simulink model "Vehicle_Model_Controller_Mar18"  (R2020b)
settings: Solver=VariableStepAuto  StartTime=0.0  StopTime=20  FixedStep=0.015  MaxStep=0.015  RelTol=1e-3
model workspace (MAT data in the model file):
  Kp = 10
  understeer_gradient = 0.05
undefined symbols (not defined in the file or in its folder): a, A1, A2, A3, b, B1, B2, B3, brakeforce_max, brakepad_mu, c, C1, C2, C3, C4, c_factor, d, DiscIntNeverNeededParam, disk_diameter, g, gearbox_efficiency, gr, I, J_z, k_limit, K_u, l, m, mech_brake, min_speed_regen, motor_efficiency, motor_limit_power, motor_limit_torque, mu_factor, P, RE, s, T, tau, tire_mu, yaw_factor
libraries: fl_lib x32, nesl_utility x24, sdl_lib x8, cstblocks x1, pid_lib x1, vehdynlibsteering x1, autolibshared x1, autolibdatasheetbattery x1
(part 2 of 3)

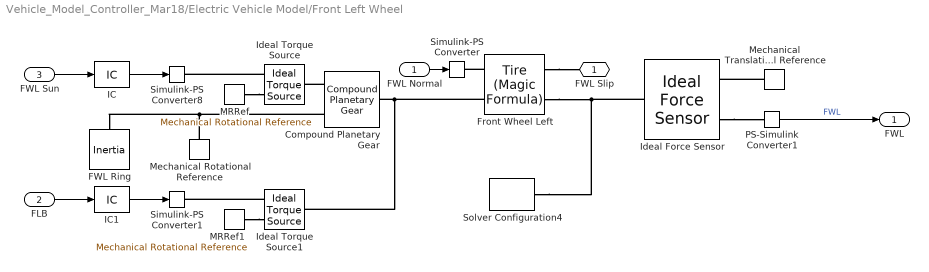
== system Vehicle_Model_Controller_Mar18/Electric Vehicle Model/Front Left Wheel ==
  FWL Normal : Inport
  FLB : Inport  Port=2
  FWL Sun : Inport  Port=3
  Compound Planetary Gear : sdl_lib/Gears/Compound Planetary Gear  rp_ratio=84/23  ps_ratio=37/24  friction_model=sdl.enum.gear_friction.constant  mu_visc=[0, 0] N*m/(rad/s)  efficiency=[.97, 1]  temperature_TLU=[280, 300, 320] K  efficiency_sp_TLU=[.95, .9, .85]  efficiency_rp_TLU=[.95, .9, .85]  pwr_thr=[.001, .001] W  thermal_mass=50 J/K  T_init=300 K  model_inertia=simscape.enum.onoff.off  planet_inertia=0.001 kg*m^2
      settings: SourceProductBaseCode=LD  InternalSimscapePortConfiguration="{\"Bottom\":[],\"Left\":[{\"id\":\"C\",\"label\":\"C\",\"type\":\"foundation.mechanical.rotational.rotational\"}],\"Right\":[{\"id\":\"R\",\"label\":\"R\",\"type\":\"foundation.mechanical.rotational.rotational\"},{\"id\":\"S\",\"label\":\"S\",\"type\":\"foundation.mechanical.rotational.rotational\"}],\"Top\":[]}"
  FWL Ring : fl_lib/Mechanical/Rotational Elements/Inertia  inertia=0.1 kg*m^2  num_ports=foundation.enum.numPorts2.one  w_specify=off  w_priority=High  w=0 rad/s  w_nominal_specify=off  w_nominal_unit=rad/s  w_nominal_value=1  t_specify=off  t_priority=None  t=0 N*m  t_nominal_specify=off  t_nominal_unit=N*m  t_nominal_value=1
  Front Wheel Left : sdl_lib/Tires & Vehicles/Tire (Magic Formula)  parameterization=sdl.enum.magic_tire_model.peak  F_z1=1400 N  F_x1=3000 N  kappa1=15  B_m=0.848  C_m=0.19  D_m=5.97  E_m=1.1  fz0=4000 N  p_Cx=1.685  p_Dx=[1.21, -.037]  p_Ex=[.344, .095, -.02, 0]  p_Kx=[21.51, -.163, .245]  p_Hx=[-.002, .002]  p_Vx=[0, 0]  v_tr_thr=0.1 m/s  r_e=0.2228169203 m  model_compliance=0  stiffness=2e5 N/m  damping=1000 N/(m/s)  model_inertia=1  inertia=0.29668158904 kg*m^2  initial_velocity=0 rad/s  model_resistance=0  resistance_model=1  coeff=0.015  p_tire=82.74e3 Pa  alpha=-0.003  beta=0.97  coeff_a=84e-4  coeff_b=6.2e-4 s/m  coeff_c=1.6e-4 s^2/m^2  v_thr=0.01 m/s
  IC : InitialCondition  Value=0
  IC1 : InitialCondition  Value=0
  Ideal Force Sensor : fl_lib/Mechanical/Mechanical Sensors/Ideal Force Sensor
  Ideal Torque Source : fl_lib/Mechanical/Mechanical Sources/Ideal Torque Source
      settings: SourceProductName=Foundation Library
  Ideal Torque Source1 : fl_lib/Mechanical/Mechanical Sources/Ideal Torque Source
      settings: SourceProductName=Foundation Library
  MRRef : fl_lib/Mechanical/Rotational Elements/Mechanical Rotational Reference
      settings: SourceProductName=Foundation Library
  MRRef1 : fl_lib/Mechanical/Rotational Elements/Mechanical Rotational Reference
      settings: SourceProductName=Foundation Library
  Mechanical Rotational Reference : fl_lib/Mechanical/Rotational Elements/Mechanical Rotational Reference
  Mechanical Translational Reference : fl_lib/Mechanical/Translational Elements/Mechanical Translational Reference
  PS-Simulink Converter1 : nesl_utility/PS-Simulink Converter  PhysicalDomain=network_engine_domain  SubClassName=ps_output  LeftPortType=input  RightPortType=output  PseudoPeriodic=off  Frequencies=[]  Unit=inherit  AffineConversion=off
      settings: SourceProductBaseCode=PW,SS
  Simulink-PS Converter : nesl_utility/Simulink-PS Converter  PhysicalDomain=network_engine_domain  SubClassName=ps_input  LeftPortType=input  RightPortType=output  PseudoPeriodic=off  Frequencies=[]  NoiseDistribution=none  NoiseParameters=[]  Unit=N  AffineConversion=off  FilteringAndDerivatives=zero  SimscapeFilterOrder=1  InputFilterTimeConstant=0.001  UdotUserProvided=0
      settings: SourceProductBaseCode=PW,SS
  Simulink-PS Converter1 : nesl_utility/Simulink-PS Converter  PhysicalDomain=network_engine_domain  SubClassName=ps_input  LeftPortType=input  RightPortType=output  PseudoPeriodic=off  Frequencies=[]  NoiseDistribution=none  NoiseParameters=[]  Unit=N*m  AffineConversion=off  FilteringAndDerivatives=zero  SimscapeFilterOrder=1  InputFilterTimeConstant=0.001  UdotUserProvided=0
      settings: SourceProductBaseCode=PW,SS
  Simulink-PS Converter8 : nesl_utility/Simulink-PS Converter  PhysicalDomain=network_engine_domain  SubClassName=ps_input  LeftPortType=input  RightPortType=output  PseudoPeriodic=off  Frequencies=[]  NoiseDistribution=none  NoiseParameters=[]  Unit=N*m  AffineConversion=off  FilteringAndDerivatives=zero  SimscapeFilterOrder=1  InputFilterTimeConstant=0.001  UdotUserProvided=0
      settings: SourceProductBaseCode=PW,SS
  Solver Configuration4 : nesl_utility/Solver Configuration  PhysicalDomain=network_engine_domain  SubClassName=solver  LeftPortType=input  RightPortType=generic  Tones=[]  Harmonics=[]  SimulateNoise=off  Profile=off  UseLocalSampling=off  EnableSwitchedLinearOptims=on  FrequencyDomain=off  UseCCode=off  RelTol=0.001  AbsTol=1e-06  MinStep=1e-09  ToWorkspace=off  RevertToSquareIcSolve=off  NumHomotopyIterations=100  PhasorMode=off  PhasorModeNumHarmonics=1  DoDC=off  ResidualTolerance=1e-09  UseLocalSolver=off  LocalSolverChoice=NE_BACKWARD_EULER_ADVANCER  LocalSolverSampleTime=0.001  DoFixedCost=off  MaxNonlinIter=200  MaxModeIter=20  ComputeImpulses=off  ImpulseIterations=20  LinearAlgebra=auto  EquationFormulation=NE_TIME_EF  DelaysMemoryBudget=1024  AutomaticFiltering=off  FilteringTimeConstant=0.1  PartitionStorageMethod=AS_NEEDED  PartitionMemoryBudget=1024  PartitionMethod=ROBUST
      settings: SourceProductBaseCode=PW,SS
  FWL Slip : PMIOPort  Side=Right
  FWL : Outport
  wires:
  PS-Simulink Converter1/1 -> FWL/1  "FWL"
  FWL Normal/1 -> Simulink-PS Converter/1
  IC/1 -> Simulink-PS Converter8/1
  FWL Sun/1 -> IC/1
  IC1/1 -> Simulink-PS Converter1/1
  FLB/1 -> IC1/1
  connections:
  Front Wheel Left/RConn1 -- FWL Slip/RConn1
  Ideal Force Sensor/RConn2 -- PS-Simulink Converter1/LConn1
  Ideal Force Sensor/LConn1 -- Front Wheel Left/RConn2 -- Solver Configuration4/RConn1
  Front Wheel Left/LConn1 -- Simulink-PS Converter/RConn1
  Mechanical Translational Reference/LConn1 -- Ideal Force Sensor/RConn1
  Mechanical Rotational Reference/LConn1 -- FWL Ring/LConn1 -- Compound Planetary Gear/RConn1
  Ideal Torque Source/RConn1 -- Simulink-PS Converter8/RConn1
  Compound Planetary Gear/RConn2 -- Ideal Torque Source/LConn1
  MRRef/LConn1 -- Ideal Torque Source/RConn2
  Ideal Torque Source1/RConn1 -- Simulink-PS Converter1/RConn1
  MRRef1/LConn1 -- Ideal Torque Source1/RConn2
  Front Wheel Left/LConn2 -- Ideal Torque Source1/LConn1 -- Compound Planetary Gear/LConn1

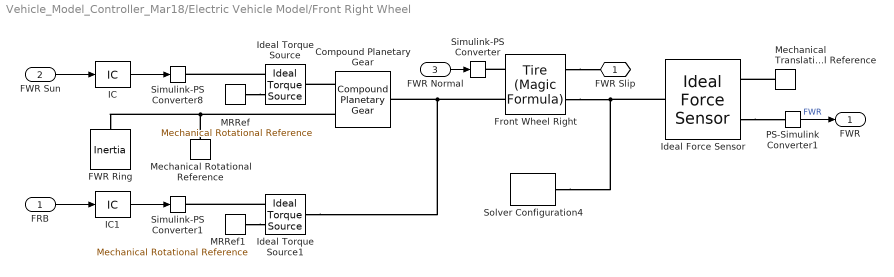
== system Vehicle_Model_Controller_Mar18/Electric Vehicle Model/Front Right Wheel ==
  FRB : Inport
  FWR Sun : Inport  Port=2
  FWR Normal : Inport  Port=3
  Compound Planetary Gear : sdl_lib/Gears/Compound Planetary Gear  rp_ratio=84/23  ps_ratio=37/24  friction_model=sdl.enum.gear_friction.constant  mu_visc=[0, 0] N*m/(rad/s)  efficiency=[.97, 1]  temperature_TLU=[280, 300, 320] K  efficiency_sp_TLU=[.95, .9, .85]  efficiency_rp_TLU=[.95, .9, .85]  pwr_thr=[.001, .001] W  thermal_mass=50 J/K  T_init=300 K  model_inertia=simscape.enum.onoff.off  planet_inertia=0.001 kg*m^2
      settings: SourceProductBaseCode=LD  InternalSimscapePortConfiguration="{\"Bottom\":[],\"Left\":[{\"id\":\"C\",\"label\":\"C\",\"type\":\"foundation.mechanical.rotational.rotational\"}],\"Right\":[{\"id\":\"R\",\"label\":\"R\",\"type\":\"foundation.mechanical.rotational.rotational\"},{\"id\":\"S\",\"label\":\"S\",\"type\":\"foundation.mechanical.rotational.rotational\"}],\"Top\":[]}"
  FWR Ring : fl_lib/Mechanical/Rotational Elements/Inertia  inertia=0.1 kg*m^2  num_ports=foundation.enum.numPorts2.one  w_specify=off  w_priority=High  w=0 rad/s  w_nominal_specify=off  w_nominal_unit=rad/s  w_nominal_value=1  t_specify=off  t_priority=None  t=0 N*m  t_nominal_specify=off  t_nominal_unit=N*m  t_nominal_value=1
  Front Wheel Right : sdl_lib/Tires & Vehicles/Tire (Magic Formula)  parameterization=sdl.enum.magic_tire_model.peak  F_z1=1400 N  F_x1=3000 N  kappa1=15  B_m=0.848  C_m=0.19  D_m=5.97  E_m=1.1  fz0=4000 N  p_Cx=1.685  p_Dx=[1.21, -.037]  p_Ex=[.344, .095, -.02, 0]  p_Kx=[21.51, -.163, .245]  p_Hx=[-.002, .002]  p_Vx=[0, 0]  v_tr_thr=0.1 m/s  r_e=0.2228169203 m  model_compliance=0  stiffness=2e5 N/m  damping=1000 N/(m/s)  model_inertia=1  inertia=0.29668158904 kg*m^2  initial_velocity=0 rad/s  model_resistance=0  resistance_model=1  coeff=0.015  p_tire=82.74e3 Pa  alpha=-0.003  beta=0.97  coeff_a=84e-4  coeff_b=6.2e-4 s/m  coeff_c=1.6e-4 s^2/m^2  v_thr=0.01 m/s
  IC : InitialCondition  Value=0
  IC1 : InitialCondition  Value=0
  Ideal Force Sensor : fl_lib/Mechanical/Mechanical Sensors/Ideal Force Sensor
  Ideal Torque Source : fl_lib/Mechanical/Mechanical Sources/Ideal Torque Source
      settings: SourceProductName=Foundation Library
  Ideal Torque Source1 : fl_lib/Mechanical/Mechanical Sources/Ideal Torque Source
      settings: SourceProductName=Foundation Library
  MRRef : fl_lib/Mechanical/Rotational Elements/Mechanical Rotational Reference
      settings: SourceProductName=Foundation Library
  MRRef1 : fl_lib/Mechanical/Rotational Elements/Mechanical Rotational Reference
      settings: SourceProductName=Foundation Library
  Mechanical Rotational Reference : fl_lib/Mechanical/Rotational Elements/Mechanical Rotational Reference
  Mechanical Translational Reference : fl_lib/Mechanical/Translational Elements/Mechanical Translational Reference
  PS-Simulink Converter1 : nesl_utility/PS-Simulink Converter  PhysicalDomain=network_engine_domain  SubClassName=ps_output  LeftPortType=input  RightPortType=output  PseudoPeriodic=off  Frequencies=[]  Unit=inherit  AffineConversion=off
      settings: SourceProductBaseCode=PW,SS
  Simulink-PS Converter : nesl_utility/Simulink-PS Converter  PhysicalDomain=network_engine_domain  SubClassName=ps_input  LeftPortType=input  RightPortType=output  PseudoPeriodic=off  Frequencies=[]  NoiseDistribution=none  NoiseParameters=[]  Unit=N  AffineConversion=off  FilteringAndDerivatives=zero  SimscapeFilterOrder=1  InputFilterTimeConstant=0.001  UdotUserProvided=0
      settings: SourceProductBaseCode=PW,SS
  Simulink-PS Converter1 : nesl_utility/Simulink-PS Converter  PhysicalDomain=network_engine_domain  SubClassName=ps_input  LeftPortType=input  RightPortType=output  PseudoPeriodic=off  Frequencies=[]  NoiseDistribution=none  NoiseParameters=[]  Unit=N*m  AffineConversion=off  FilteringAndDerivatives=zero  SimscapeFilterOrder=1  InputFilterTimeConstant=0.001  UdotUserProvided=0
      settings: SourceProductBaseCode=PW,SS
  Simulink-PS Converter8 : nesl_utility/Simulink-PS Converter  PhysicalDomain=network_engine_domain  SubClassName=ps_input  LeftPortType=input  RightPortType=output  PseudoPeriodic=off  Frequencies=[]  NoiseDistribution=none  NoiseParameters=[]  Unit=N*m  AffineConversion=off  FilteringAndDerivatives=zero  SimscapeFilterOrder=1  InputFilterTimeConstant=0.001  UdotUserProvided=0
      settings: SourceProductBaseCode=PW,SS
  Solver Configuration4 : nesl_utility/Solver Configuration  PhysicalDomain=network_engine_domain  SubClassName=solver  LeftPortType=input  RightPortType=generic  Tones=[]  Harmonics=[]  SimulateNoise=off  Profile=off  UseLocalSampling=off  EnableSwitchedLinearOptims=on  FrequencyDomain=off  UseCCode=off  RelTol=0.001  AbsTol=1e-06  MinStep=1e-09  ToWorkspace=off  RevertToSquareIcSolve=off  NumHomotopyIterations=100  PhasorMode=off  PhasorModeNumHarmonics=1  DoDC=off  ResidualTolerance=1e-09  UseLocalSolver=off  LocalSolverChoice=NE_BACKWARD_EULER_ADVANCER  LocalSolverSampleTime=0.001  DoFixedCost=off  MaxNonlinIter=200  MaxModeIter=20  ComputeImpulses=off  ImpulseIterations=2  LinearAlgebra=auto  EquationFormulation=NE_TIME_EF  DelaysMemoryBudget=1024  AutomaticFiltering=off  FilteringTimeConstant=0.001  PartitionStorageMethod=AS_NEEDED  PartitionMemoryBudget=1024  PartitionMethod=ROBUST
      settings: SourceProductBaseCode=PW,SS
  FWR Slip : PMIOPort  Side=Right
  FWR : Outport
  wires:
  PS-Simulink Converter1/1 -> FWR/1  "FWR"
  FWR Normal/1 -> Simulink-PS Converter/1
  IC/1 -> Simulink-PS Converter8/1
  FWR Sun/1 -> IC/1
  IC1/1 -> Simulink-PS Converter1/1
  FRB/1 -> IC1/1
  connections:
  Front Wheel Right/RConn1 -- FWR Slip/RConn1
  Front Wheel Right/LConn1 -- Simulink-PS Converter/RConn1
  Ideal Force Sensor/RConn2 -- PS-Simulink Converter1/LConn1
  Ideal Force Sensor/LConn1 -- Front Wheel Right/RConn2 -- Solver Configuration4/RConn1
  Mechanical Translational Reference/LConn1 -- Ideal Force Sensor/RConn1
  MRRef/LConn1 -- Ideal Torque Source/RConn2
  Compound Planetary Gear/RConn2 -- Ideal Torque Source/LConn1
  Ideal Torque Source/RConn1 -- Simulink-PS Converter8/RConn1
  Ideal Torque Source1/LConn1 -- Front Wheel Right/LConn2 -- Compound Planetary Gear/LConn1
  Mechanical Rotational Reference/LConn1 -- FWR Ring/LConn1 -- Compound Planetary Gear/RConn1
  Ideal Torque Source1/RConn1 -- Simulink-PS Converter1/RConn1
  MRRef1/LConn1 -- Ideal Torque Source1/RConn2

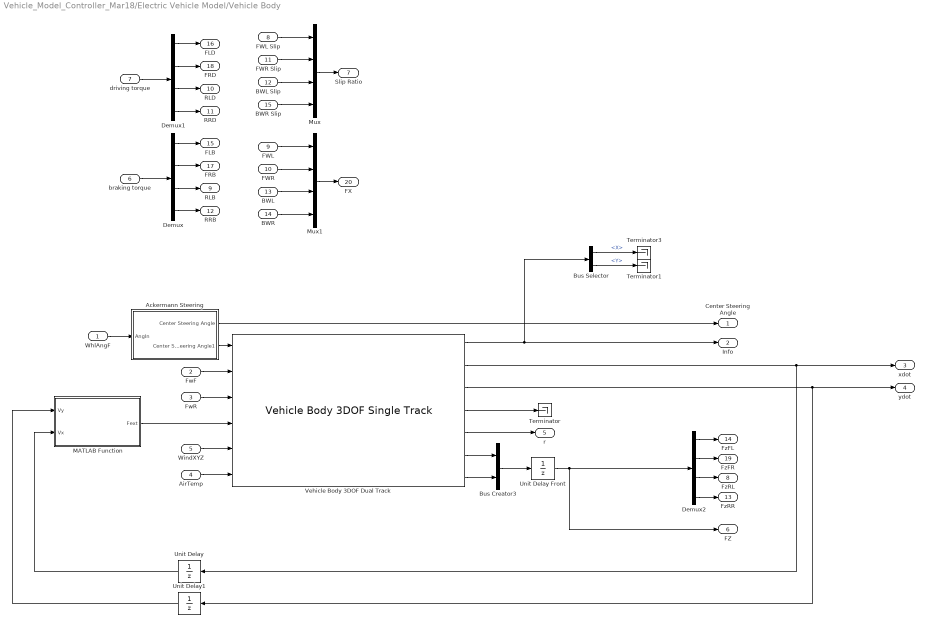
== system Vehicle_Model_Controller_Mar18/Electric Vehicle Model/Vehicle Body ==
  WhlAngF : Inport
  FwF : Inport  Port=2
  FwR : Inport  Port=3
  AirTemp : Inport  Port=4
  WindXYZ : Inport  Port=5
  braking torque : Inport  Port=6
  driving torque : Inport  Port=7
  FWL Slip : Inport  Port=8
  FWL : Inport  Port=9
  FWR : Inport  Port=10
  FWR Slip : Inport  Port=11
  BWL Slip : Inport  Port=12
  BWL : Inport  Port=13
  BWR : Inport  Port=14
  BWR Slip : Inport  Port=15
  Ackermann Steering : Subsystem
  Bus Creator3 : BusCreator  Inputs=2
  Bus Selector : BusSelector  OutputSignals=InertFrm.Cg.Disp.X,InertFrm.Cg.Disp.Y
  Demux : Demux
  Demux1 : Demux
  Demux2 : Demux
  MATLAB Function : MATLAB Function  TreatAsAtomicUnit=on
  Mux : Mux
  Mux1 : Mux
  Terminator : Terminator
  Terminator1 : Terminator
  Terminator3 : Terminator
  Unit Delay : UnitDelay  SampleTime=-1  HasFrameUpgradeWarning=on
  Unit Delay Front : UnitDelay  InitialCondition=[547 547 547 547]  SampleTime=-1  HasFrameUpgradeWarning=on
  Unit Delay1 : UnitDelay  SampleTime=-1  HasFrameUpgradeWarning=on
  Vehicle Body 3DOF Dual Track : autolibshared/Vehicle Body 3DOF Single Track  trackMode=Dual  inputMode=External forces  frontSteerMode=on  rearSteerMode=off  windMode=on  muMode=off  extFMode=on  extMMode=off  htchFMode=off  htchMMode=off  extXo=off  extpsio=off  extxdoto=off  extro=off  extYo=off  extTamb=on  extydoto=off  aMode=2  NF=2  NR=2  m=308  a=0.7922471  b=0.7828529  h=0.295  dh=1  hh=0.2  X_o=0  xdot_o=0  CalphaMode=off  sigmaMode=on  d=0  hl=0  w=[1.29579,1.24204]  Cy_f=25e3  Cy_r=25e3  sigma_f=.1  sigma_r=.1  alpha_f_brk=[-.1 .1]  Cy_f_data=[-9e3 9e3]  alpha_r_brk=[-.1 .1]  Cy_r_data=[-9e3 9e3]  Y_o=0  ydot_o=0  Izz=75  psi_o=0  r_o=0  Af=1.0221  Cd=1.149  Cl=0  Cpm=.000001  beta_w=[0:0.01:0.3]  Cs=[0:0.03:0.9]  Cym=[0:0.01:0.3]  Pabs=101325  Tair=273  g=9.81  mu=1  xdot_tol=.1  Fznom=15000  Fxtire_sat=7e4  Fytire_sat=7e4  longOff=0  latOff=0  vertOff=0  wrapAng=off
      settings: SourceProductBaseCode=PW,DR,MT,UV,VE
  Center Steering Angle : Outport
  Info : Outport  Port=2
  xdot : Outport  Port=3
  ydot : Outport  Port=4
  r : Outport  Port=5
  FZ : Outport  Port=6
  Slip Ratio : Outport  Port=7
  FzRL : Outport  Port=8
  RLB : Outport  Port=9
  RLD : Outport  Port=10
  RRD : Outport  Port=11
  RRB : Outport  Port=12
  FzRR : Outport  Port=13
  FzFL : Outport  Port=14
  FLB : Outport  Port=15
  FLD : Outport  Port=16
  FRB : Outport  Port=17
  FRD : Outport  Port=18
  FzFR : Outport  Port=19
  FX : Outport  Port=20
  wires:
  Vehicle Body 3DOF Dual Track/3 -> ydot/1, Unit Delay1/1
  Vehicle Body 3DOF Dual Track/1 -> Bus Selector/1, Info/1
  AirTemp/1 -> Vehicle Body 3DOF Dual Track/6
  Vehicle Body 3DOF Dual Track/4 -> Terminator/1
  Vehicle Body 3DOF Dual Track/5 -> r/1
  WindXYZ/1 -> Vehicle Body 3DOF Dual Track/5
  Demux2/1 -> FzFL/1
  Demux2/2 -> FzFR/1
  Demux2/3 -> FzRL/1
  Demux2/4 -> FzRR/1
  Ackermann Steering/1(Center Steering Angle) -> Center Steering Angle/1
  WhlAngF/1 -> Ackermann Steering/1(AngIn)
  Bus Selector/1 -> Terminator3/1  "<X>"
  Bus Selector/2 -> Terminator1/1  "<Y>"
  Vehicle Body 3DOF Dual Track/7 -> Bus Creator3/2
  Vehicle Body 3DOF Dual Track/6 -> Bus Creator3/1
  Bus Creator3/1 -> Unit Delay Front/1
  MATLAB Function/1(Fext) -> Vehicle Body 3DOF Dual Track/4
  Unit Delay/1 -> MATLAB Function/2(Vx)
  Unit Delay1/1 -> MATLAB Function/1(Vy)
  Vehicle Body 3DOF Dual Track/2 -> xdot/1, Unit Delay/1
  FWL Slip/1 -> Mux/1
  BWR Slip/1 -> Mux/4
  FWR Slip/1 -> Mux/2
  BWL Slip/1 -> Mux/3
  Mux/1 -> Slip Ratio/1
  Ackermann Steering/2(Center Steering Angle1) -> Vehicle Body 3DOF Dual Track/1
  FwR/1 -> Vehicle Body 3DOF Dual Track/3
  FwF/1 -> Vehicle Body 3DOF Dual Track/2
  Demux/3 -> RLB/1
  Demux/1 -> FLB/1
  Demux/2 -> FRB/1
  Demux/4 -> RRB/1
  Demux1/3 -> RLD/1
  Demux1/1 -> FLD/1
  Demux1/4 -> RRD/1
  Demux1/2 -> FRD/1
  braking torque/1 -> Demux/1
  FWL/1 -> Mux1/1
  FWR/1 -> Mux1/2
  BWR/1 -> Mux1/4
  BWL/1 -> Mux1/3
  driving torque/1 -> Demux1/1
  Unit Delay Front/1 -> Demux2/1, FZ/1
  Mux1/1 -> FX/1

== system Vehicle_Model_Controller_Mar18/Motor and Battery/Motors ==
  Battery Voltage : Inport
  ang_vel_RAD : Inport  Port=2
  Torque Request : Inport  Port=3
  " " : MATLAB Function  TreatAsAtomicUnit=on
  "  " : MATLAB Function  TreatAsAtomicUnit=on
  Gain : Gain  Gain=9.5492965964254
  Battery Current : Outport
  Battery Power : Outport  Port=2
  Motor Torque : Outport  Port=3
  wires:
  Torque Request/1 -> " "/2(torque_request)
  Battery Voltage/1 -> "  "/1(Battery_Voltage)
  ang_vel_RAD/1 -> Gain/1, "  "/2(ang_vel_RAD)
  "  "/1(battery_current) -> Battery Current/1
  " "/1(motor_torque) -> Motor Torque/1, "  "/3(Motor_torque)
  "  "/2(battery_power) -> Battery Power/1
  Gain/1 -> " "/1(ang_vel_RPM)

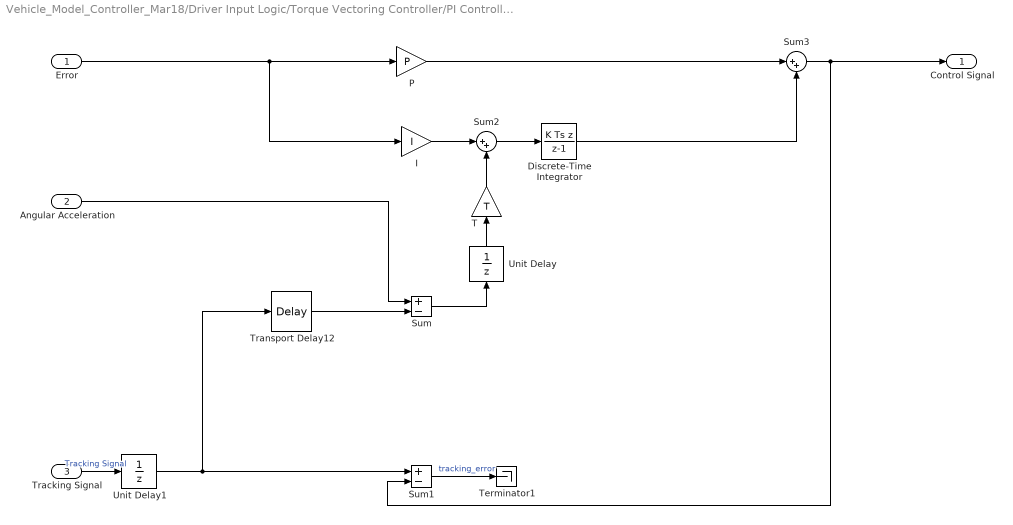
== system Vehicle_Model_Controller_Mar18/Driver Input Logic/Torque Vectoring Controller/PI Controller ==
  Error : Inport
  Angular Acceleration : Inport  Port=2
  Tracking Signal : Inport  Port=3
  Discrete-Time Integrator : DiscreteIntegrator  IntegratorMethod=Integration: Backward Euler  gainval=1  SampleTime=-1  ICPrevOutput=DiscIntNeverNeededParam  ICPrevScaledInput=DiscIntNeverNeededParam
  I : Gain  Gain=I
  P : Gain  Gain=P
  Sum : Sum  Inputs=+-
  Sum1 : Sum  Inputs=+-
  Sum2 : Sum  Inputs=|++
  Sum3 : Sum  Inputs=|++
  T : Gain  Gain=T
  Terminator1 : Terminator
  Transport Delay12 : TransportDelay  DelayTime=0.022  BufferSize=25000
  Unit Delay : UnitDelay  SampleTime=-1  HasFrameUpgradeWarning=on
  Unit Delay1 : UnitDelay  SampleTime=-1  HasFrameUpgradeWarning=on
  Control Signal : Outport
  wires:
  P/1 -> Sum3/1
  Unit Delay/1 -> T/1
  T/1 -> Sum2/2
  I/1 -> Sum2/1
  Sum2/1 -> Discrete-Time Integrator/1
  Discrete-Time Integrator/1 -> Sum3/2
  Sum1/1 -> Terminator1/1  "tracking_error"
  Sum/1 -> Unit Delay/1
  Error/1 -> I/1, P/1
  Transport Delay12/1 -> Sum/2
  Angular Acceleration/1 -> Sum/1
  Sum3/1 -> Control Signal/1, Sum1/2
  Unit Delay1/1 -> Transport Delay12/1, Sum1/1
  Tracking Signal/1 -> Unit Delay1/1  "Tracking Signal"

== system Vehicle_Model_Controller_Mar18/Electric Vehicle Model/Vehicle Body/Ackermann Steering ==
  AngIn : Inport
  Deg to Rad : Gain  Gain=pi/180
  Kinematic Steering : vehdynlibsteering/Kinematic Steering  StrgType=Ackerman  StrgRatioType=Constant  Loc=Front  NrmlFctr=0.1  TrckWdth=1.29579  WhlBase=1.5751  Db=0  StrgRng=pi/6  StrgAngBpts="[-6.2832   -5.0265   -3.7699   -2.5133   -1.2566         0    1.2566    2.5133    3.7699    5.0265    6.2832]"  StrgRatioTbl=|  StrgRatio=1  StrgArmLngth=0.1  RckCsLngth=0.5  TieRodLngth=0.248  D=0.2  PnnRadius=0.0057  PnnRadiusTbl="[0.0055    0.0055    0.0056    0.0057    0.0058    0.0057    0.0057    0.0057    0.0056    0.0055    0.0055]"  RodLngth=0.1  ParaArmLngth=0.9  aMode=2
      | [13.5000   13.3750   13.2500   13.1250   13.0000   13.0000   13.0000   13.1250   13.2500   13.3750   13.5000
      | ]
  Mux : Mux  Inputs=2
  Mux3 : Mux  Inputs=2
  Terminator : Terminator
  Terminator1 : Terminator
  Center Steering Angle : Outport
  Center Steering Angle1 : Outport  Port=2
  wires:
  Kinematic Steering/2 -> Mux3/1
  Kinematic Steering/3 -> Mux3/2
  Kinematic Steering/1 -> Terminator/1
  Deg to Rad/1 -> Mux/1, Mux/2, Center Steering Angle/1, Kinematic Steering/1  "steering_angle"
  AngIn/1 -> Deg to Rad/1  "steering_angle"
  Mux3/1 -> Terminator1/1  "ackermann angles"
  Mux/1 -> Center Steering Angle1/1

== matlab function Vehicle_Model_Controller_Mar18/Driver Input Logic/Torque Vectoring Controller/Layer 1 ==
  data: driver_input output; power_limits_battery output; acker_steer_angles output; FY output; omega_w output; T2F output single size=[1 4]; T_brake output size=[1 4]; yaw output; yaw_ref output size=[1 2]; driver_input input; power_limits_battery input; C input; omega_w input; center_steer_angle input; acker_steer_angles input; FY input size=[1 4]; Vg input; yaw input; K_u parameter; gr parameter; gearbox_efficiency parameter; tau parameter; c_factor parameter; J_z parameter; l parameter; s parameter; RE parameter; g parameter; tire_mu parameter; brakeforce_max parameter; brakepad_mu parameter; disk_diameter parameter; mech_brake parameter; yaw_factor parameter; m parameter
function [driver_input, power_limits_battery, acker_steer_angles, FY, omega_w, T2F, T_brake, yaw, yaw_ref] = Layer_1(driver_input, power_limits_battery, C,omega_w, center_steer_angle, acker_steer_angles, FY, Vg, yaw, K_u, gr, gearbox_efficiency, tau, c_factor, J_z, l, s, RE, g, tire_mu, brakeforce_max, brakepad_mu, disk_diameter, mech_brake, yaw_factor, m)
%% Layer 1 Computation
% Developer(s):    David Farell
%                  Demetrius Gulewicz
%                  Elliot Stockwell
%                  Tao Sun
%
% Developed for: Purdue Electric Racing
% Date:          12/25/2021
%
% Description: This function primarily computes the reference yaw rate, 
%              and the brake forces & distribution.
%
%
%% Pass Through Signals
% driver_input - Proportion Of Total Available Power To Use [Unitless][1x1]
% power_limits_battery - Max & Min Total Battery Power Output [W][2x1]
% center_steer_angle - Steering Column Angle From Neutral [rad][1x1]
% acker_steer_angles - Angle Tires Are Turned From Neutral [rad][2x1]
% FY - Tires Forces y Direction, Tire Fixed Coordinates [N][1x4]
% omega_w - Angular Velocity Of Tires, Tire Fixed Coordinates [m/s][1x4]
% yaw - Yaw Rate z Direction, Vehicle Fixed Coordinates  [rad/s][1x1]
%
%
%% Input Only
% Vg - Center Of Gravity Velocity, Vehicle Fixed Coordinates [m/s][1x2]
%
%
%% Output Only
% T2F - Convert Torque At The Motor Shaft to Force At The Tire [1/m][1x4]
% T_brake - Mechanical Brake Torque On Each Tire [Nm][1x4]
% yaw_ref - The Desired & Max Allowed Yaw Rate [rad/s][1x2]
%
%
%% Constants
% global g; % Acceleration Due To Gravity [m/s^2][1x1]
% global tire_mu; % Maximum Friction Coefficient [Unitless][1x1]
% global gr; % Gear ratios [Unitless][1x4]
% global gearbox_efficiency; % Gearbox Power Transmission Efficiency [Unitless][1x4]
% global r; % Tire Radius [m][1x1]
% global l; % Wheelbase [m][1x2]
% global K_u; % Understeer Gradient [rad/m/s^2][1x1]
% global c_factor; % Max Yaw Equation Contributing Factor [Unitless][1x1]
% global brakeforce_max; % Max Force Brakes Can Exert On Each Tire Axle [N][1x4]
% global brakepad_mu; % Brakepad Friction Coefficient[Unitless][1x1]
% global mech_brake; % Value Of driver_input Where Mechanical Braking Begins [Unitless][1x1]
% global disk_diameter; % Diameter of brake disk [m][1x1]
% global yaw_factor; % Coefficent to adjust desired yaw magnitude [1x1]


%% Calculation
% Convert Torque At The Motor Shaft to Force At The Wheel
% During Runtime, T2F Is Constant
T2F = single((gr .* gearbox_efficiency) ./ RE);
T2F = single([29 29 34.772 34.772]);

% Compute Ku, the understeer gradient
gen_coeff = (m / sum(l));
corner_1 = l(2) / sum(C(1:2));
corner_2 = (l(1) / sum(C(3:4)));

Ku = gen_coeff * (corner_1 - corner_2);


% Yaw Calculations
% If yaw_des or yaw_max ever exceed 2, then the exact value is no longer
% needed. As in, the ceiling of these two variables is 2.
v_cog = norm(Vg);
yaw_des = (yaw_factor * v_cog * center_steer_angle) / ((l(1) + l(2)) + (Ku * v_cog ^ 2));
yaw_max = (c_factor * tire_mu * g) / (v_cog);

% Control For Large Max Yaw, For Better Viewing
if yaw_max > 3
    yaw_max = 3;
end

yaw_ref = [yaw_des, yaw_max];

% Apply correct sign convention to yaw_ref
if center_steer_angle < 0
    yaw_ref(2) = -yaw_ref(2);
end

% Compute brake force and distribution
% for small brakes (input >= mech_brake), only regen braking
% for large brakes (input <= mech_brake), regen & mechanical braking
% note: actual force may not be proportional to the input
T_brake = [0,0,0,0];

if driver_input <= mech_brake   
    brakeforce_ratio = [1, 1, 1, 1] .* -(driver_input - mech_brake) / (1 + mech_brake);
    T_brake = -1.*brakeforce_ratio.*brakeforce_max.*brakepad_mu.*disk_diameter;
    driver_input = -1;
end

if Vg(1) < 0
    T_brake = -T_brake;
end

if abs(Vg(1)) < 0.1
   T_brake = [0 0 0 0]; 
end

if driver_input <= 0 && driver_input >= mech_brake
    driver_input = -driver_input / mech_brake;  % in scale of [-1,0]
end

end

== matlab function Vehicle_Model_Controller_Mar18/Driver Input Logic/Torque Vectoring Controller/Layer 2 ==
  data: driver_input output; power_limit_battery output; FY output; omega_m output size=[1 4]; x output size=[1 4]; y output size=[1 4]; T2F output; slip_limit output; torque_limit_motor output; tau_limit_upper output; tau_limit_lower output; rpm_limit output; prev_torque input; driver_input input; power_limits_battery input; acker_steer_angles input; FY input; omega_w input; T2F input; T_brake input; yaw input; yaw_ref input; Fx_max input; yaw_err output; motor_limit_power parameter; motor_efficiency parameter; J_z parameter; gr parameter; RE parameter; tau parameter; motor_limit_torque parameter; t parameter; l parameter; disk_diameter parameter; s parameter
function [driver_input, power_limit_battery, FY, omega_m, x, y, T2F, slip_limit, torque_limit_motor, tau_limit_upper, tau_limit_lower, rpm_limit, yaw_err] = Layer_2(prev_torque, driver_input, power_limits_battery, acker_steer_angles, FY, omega_w, T2F, T_brake, yaw, yaw_ref,Fx_max, motor_limit_power, motor_efficiency, J_z, gr, RE, tau, motor_limit_torque, t, l, disk_diameter, s)
%% Layer 2 Computation
% Developer(s):    David Farell
%                  Demetrius Gulewicz
%                  Elliot Stockwell
%                  Tao Sun
%
% Developed for: Purdue Electric Racing
% Date:          12/25/2021
%
% Description: This function primarily computes the maximum and minimum
%              torque that can be requested, based on slip, power, and 
%              transient constraints. Also computes yaw error.
%
%
%% Pass Through Signals
% prev_torque - Torque requested to motor in previous time step [Nm][4x1]
% driver_input - Proportion Of Total Available Power To Use [Unitless][1x1]
% T2F - Convert Torque At The Motor Shaft to Force At The Tire [1/m][1x4]
% FY - Tires Forces y Direction, Tire Fixed Coordinates [N][4x1]
%
%
%% Input Only
% power_limits_battery - Max & Min Total Battery Power Output [W][2x1]
% center_steer_angle - Steering Column Angle From Neutral [rad][1x1]
% acker_steer_angles - Angle Tires Are Turned From Neutral [rad][2x1]
% Fx_max - Max Tire Forces x Direction, Tire Fixed Coordinates [N][1x4]
% omega_w - Angular Velocity Of Tires, Tire Fixed Coordinates [m/s][1x4]
% yaw - Yaw Rate z Direction, Vehicle Fixed Coordinates  [rad/s][1x1]
% T_brake - Mechanical Brake Torque On Each Tire [Nm][1x4]
% yaw_ref - The Desired & Max Allowed Yaw Rate [rad/s][1x2]
%
%
%% Output Only
% power_limit_battery - Max OR Min Total Battery Power Output [W][1x1]
% omega_m - Motor Shaft Angular Velocity [rad/s][1x4]
% x - Equivalent Distances That Fx Acts From CoG [m][1x4]
% y - Equivalent Distances That Fy Acts From CoG [m][1x4] 
% slip_limit - Max Torque Before Tire Slips [Nm][1x4]
% torque_limit_motor - Max Torque Motor Can Output [Nm][1x4]
% tau_limit_upper - Max Torque Motor Is Allowed To Change To [Nm][1x4]
% tau_limit_lower - Min Torque Motor Is Allowed To Change To [Nm][1x4]
% yaw_err - Error Between Target & Actual Yaw Rate [rad/s][1x1]
% RPM_limit - Max Torque Possible at Current RPM [Nm][1x4]
%
%
%% Constants
% global s; % Half track width [m][1x2]
% global l; % Wheelbase [m][1x2]
% global motor_limit_power; % Absolute Power Limit For Each Motor [W][1x4]
% global motor_efficiency; % Motor Efficiency [Unitless][1x4]
% global tau; % Motor Response Time Constant [s][1x1]
% global t; % Controller Timing [s][1x1]
% global gr; % Gear Ratios [Unitless][1x4]
% global r; % Tire Radius [m][1x1]
% global motor_limit_torque; % Min & Max Torque Request From Motor [Nm][1x2]


%% Yaw Error
% Calculate the Yaw Error, Apply Sign Convention
if yaw_ref(1) == 0 && yaw(1) == 0
    yaw_err = 0;
else
    min_yaw_ref = sign(yaw_ref(1)) * min(abs(yaw_ref));
    yaw_err = (min_yaw_ref - yaw);
end

%% Moment Arm For Tire Forces
% Calculate K_1 Vehicle Constants
x_1 = (s(1) * cos(acker_steer_angles(1))) + (l(1) * sin(acker_steer_angles(1)));
x_2 = (-1 * s(1) * cos(acker_steer_angles(2))) + (l(1) * sin(acker_steer_angles(2)));
x_3 = s(2);
x_4 = -s(2);
x = [x_1, x_2, x_3, x_4]; 

% Calculate K_2 Vehicle Constants
y_1 = (-1 * s(1) * sin(acker_steer_angles(1))) + (l(1) * cos(acker_steer_angles(1)));    
y_2 = (s(1) * sin(acker_steer_angles(2))) + (l(1) * cos(acker_steer_angles(2)));
y_3 = -l(2);
y_4 = -l(2);
y = [y_1, y_2, y_3, y_4]; 


%% Slip Limit
% Calculate Torque Limit Due to Power and Slip
slip_limit = (Fx_max-(T_brake./RE)) ./ T2F; 


%% Power Limit
% Motor Shaft Speed, RAD/S
omega_m = omega_w .* gr;

% % If torque_limit_motor ever exceed 30, then the exact value is no longer
% needed. As in, the ceiling is 30
torque_limit_motor = (motor_limit_power .* motor_efficiency) ./ omega_m;

% Erase power limit solution above torque limit, for better data
% visualization
for i = 1:4
    if torque_limit_motor(i) > 25 
        torque_limit_motor(i) = 25;
    elseif torque_limit_motor(i) < -25 && omega_m(i) > 0
        torque_limit_motor(i) = -0.01; 
    elseif torque_limit_motor(i) < -25 && omega_m(i) < 0
        torque_limit_motor(i) = 25; 
    end
end


%% RPM Limit
% This section in practice will probably just be a lookup table, when PER
% gets the chance to get test results for the motors
% Motor Shaft Speed, rpm
ang_vel_RPM = omega_m .* 9.5492965964254;

% quadratic constants that connect current and max RPM of motors
a_v = 0.2667;
b_v = -66.353;
c_v = 10452 - ang_vel_RPM;

% quadratic constants that connnect current and max torque of motors
a_t = -0.0987;
b_t = 45.799;
c_t = -129.65;

% maximum possible current at the current RPM
max_current = [0, 0, 0, 0];

% calculate the maximum current possible at the current RPM
for i = [1:4]
   if ang_vel_RPM(i) < 7000
       max_current(i) = 70;
   else
       max_current(i) = (-b_v - sqrt(b_v^2 - (4*a_v.*c_v(i)))) .* (1/(2*a_v));
   end
end

% calculate the maximum torque at the max current
rpm_limit = ((a_t .* (max_current.^2)) + (b_t .* max_current) + c_t) ./ 100;
for i = [1:4]
   if rpm_limit(i) < 0
      rpm_limit(i) = 0;
   end
end


%% Motor Response Limit
% Calculate Constants for getting limit on motor output torque due to
% motor response time
% Note: e_term, c_lower, c_upper are based on tunable parameters, during
% runtime, they are constant
e_term = exp(-t / tau);
c_lower = (1 - e_term) .* motor_limit_torque(1);
c_upper = (1 - e_term) .* motor_limit_torque(2);
c_constant = (prev_torque .* e_term)';

% Max and Min Torque Limits due to motor response time
tau_limit_upper = max([c_upper + c_constant; c_constant + .01]);
tau_limit_lower = min([c_lower + c_constant; c_constant - .01]);

% If driver is not pressing acceleration pedal, no positive torque is allowed
if driver_input <= 0
%    tau_limit_upper = [0, 0, 0, 0];
   power_limit_battery = power_limits_battery(2);  
else
    power_limit_battery = power_limits_battery(1);
end

end

== matlab function Vehicle_Model_Controller_Mar18/Electric Vehicle Model/Vehicle Body/MATLAB Function ==
  data: Vy input; Vx input; Fext output
function Fext = get_downforce(Vy, Vx)
%% Constants
rho = 1.225; % Air density [Kg/m^3]
cl = 2.11014; % Lift coefficient [unitless]
A = 1.0221; % Frontal Area [m^2]


%% Computation
% Compute CoG Velocity
Vcog = Vx^2 + Vy^2;

% Compute DownForce
Fz = 0.5 * rho * Vcog * cl * A;
Fext = [0, 0, Fz];

== matlab function Vehicle_Model_Controller_Mar18/Motor and Battery/Motors/  ==
  data: ang_vel_RPM input; motor_torque output size=[1 4]; torque_request input
function motor_torque = get_torque(ang_vel_RPM, torque_request)
%% Actual Torque Output
% Developers:    Demetrius Gulewicz

% Developed for: Purdue Electric Racing
% Date:          09/18/2021
%
% Definitions:
% ang_vel:   Angular velocity of each wheel on the wheel fixed y axis [RPM]
% torque_request: Requested torque from the LP model                  [Nm]

%% Constants
% quadratic constants that connect current and max RPM of motors
a_v = 0.2667;
b_v = -66.353;
c_v = 10452 - ang_vel_RPM;

% quadratic constants that connnect current and max torque of motors
a_t = -0.0987;
b_t = 45.799;
c_t = -129.65;

% maximum possible current at the current RPM
max_current = [0, 0, 0, 0];


%% Calculate Maximum Torque Possible
% calculate the maximum current possible at the current RPM
for i = [1:4]
   if ang_vel_RPM(i) < 7000
       max_current(i) = 70;
   else
       max_current(i) = (-b_v - sqrt(b_v^2 - (4*a_v.*c_v(i)))) .* (1/(2*a_v));
   end
end

% calculate the maximum torque at the max current
max_torque = (a_t .* (max_current.^2)) + (b_t .* max_current) + c_t;
for i = [1:4]
   if max_torque(i) < 0
      max_torque(i) = 0;
   end
end

motor_torque_matrix = [max_torque; torque_request'];
motor_torque = min(motor_torque_matrix);

== matlab function Vehicle_Model_Controller_Mar18/Driver Input Logic/Torque Vectoring Controller/Layer 0 ==
  settings: updateMethod=DISCRETE
  data: C output; omega_w input; center_steer_angle input; Vx input; Vy input; yaw input; FZ input size=[1 4]; SL input size=[1 4]; omega_w output; center_steer_angle output; acker_steer_angles output; FY output; Vg output; yaw output; Fx_max output; RE parameter; s parameter; l parameter; vel input; mu_factor parameter; k_limit parameter; A1 parameter; A2 parameter; A3 parameter; B1 parameter; B2 parameter; B3 parameter; C2 parameter; C1 parameter; C3 parameter; C4 parameter; a parameter; b parameter; c parameter; d parameter
function [C,omega_w,center_steer_angle,acker_steer_angles,FY,Vg,yaw,Fx_max]  = Layer_0(omega_w,center_steer_angle,Vx,Vy,yaw,FZ,SL,RE, s, l, vel, mu_factor, k_limit, A1, A2, A3, B1, B2, B3, C2, C1, C3, C4, a, b, c, d)
%% Pass Through Signals
% center_steer_angle - Steering Column Angle From Neutral [rad][1x1]
% omega_w - Angular Velocity Of Tires, Tire Fixed Coordinates [m/s][1x4]
% yaw - Yaw Rate z Direction, Vehicle Fixed Coordinates  [rad/s][1x1]
%
%
%% Input Only
% shock_pot_disp - [mm][1x4]
% Vx - Center Of Gravity x Velocity, Vehicle Fixed Coordinates [m/s][1x1]
% Vy - Center Of Gravity y Velocity, Vehicle Fixed Coordinates [m/s][1x1]
% vel - Axle Velocity at Each Tire [m/s][1x6]
% SL - Slip Ratio from Tire Block [Unitless][1x4]
%
%
%% Output Only
% acker_steer_angles - Angle Tires Are Turned From Neutral [rad][2x1]
% Fx_max - Max Tire Forces x Direction, Tire Fixed Coordinates [N][1x4]
% FY - Tires Forces y Direction, Tire Fixed Coordinates [N][1x4]
% Vg - Center Of Gravity Velocity, Vehicle Fixed Coordinates [m/s][1x2]
%
%
%% Constants
% global s; % Half track width [m][1x2]
% global l; % Wheelbase [m][1x2]
% global RE; % Effective Radius of tire [m][1x1]
% global mu_factor; % Coefficient of Friction Modifier
% global k_limit; % Max Combined Slip before problems happen


%% Compute FY & FZ
% Incomplete
for i = 1:4
    if ~(isfinite(1/FZ(i)))
        FZ(i) = 1;
    end
end

%% Compute Steering Angles
% Incomplete
acker_steer_angles = [center_steer_angle center_steer_angle];


%% Simulation Only
% This section is only for simulation. IGNORE THIS SECTION
% Motor Shaft Speed, m/s
v_fl = (vel(1) * cos(acker_steer_angles(1))) + (vel(2) * sin(acker_steer_angles(1)));
v_fr = (vel(3) * cos(acker_steer_angles(2))) + (vel(4) * sin(acker_steer_angles(2)));
v_rl = vel(5);
v_rr = vel(6);
v_w = [v_fl v_fr v_rl v_rr];

% Motor Shaft Speed, Rad/s
omega_w = ((SL .* abs(v_w)) + v_w) ./ RE;

%% Compute Tire Slip
% Velocity at CoG
Vg = [Vx Vy];

% Velocity at each Tire
V_fl = Vg + (yaw .* [s(1) l(1)]);
V_fr = Vg + (yaw .* [-s(1) l(1)]);
V_rl = Vg + (yaw .* [s(2) -l(2)]);
V_rr = Vg + (yaw .* [-s(2) -l(2)]);

V = [V_fl V_fr V_rl V_rr];

% Individual slip angles, it blows up at low velocity
if abs(Vg(1)) > 0.1
    phi_fl = atan2(V_fl(2), V_fl(1));
    phi_fr = atan2(V_fr(2), V_fr(1));
    phi_rl = atan2(V_rl(2), V_rl(1));
    phi_rr = atan2(V_rr(2), V_rr(1));
else
    phi_fl = 0;
    phi_fr = 0;
    phi_rl = 0;
    phi_rr = 0;
end

phi = [phi_fl phi_fr phi_rl phi_rr];

% Compute Slip Angle
SA_fl = -phi_fl + acker_steer_angles(1);
SA_fr = -phi_fr + acker_steer_angles(2);
SA_rl = -phi_rl;
SA_rr = -phi_rr;

SA = [SA_fl SA_fr SA_rl SA_rr];

% Compute Slip Ratio
SL_fl = ((RE * omega_w(1))/(norm(V_fl) * cos(SA_fl))) - 1;
SL_ff = ((RE * omega_w(2))/(norm(V_fr) * cos(SA_fr))) - 1;
SL_rl = ((RE * omega_w(3))/(norm(V_rl) * cos(SA_rl))) - 1;
SL_rr = ((RE * omega_w(4))/(norm(V_rr) * cos(SA_rr))) - 1;

% This line is commented out only for simulation. On this vehicle, this
% line is to be included.
% SL = [SL_fl SL_ff SL_rl SL_rr];

%% Non Dimensional Tire Model
% C model
FZ_C = [0 204.13 427.04 668.1 895.72 1124.40 1324.40];
C_param = [0 13757.41 21278.97 26666.02 30253.47 30313.18 30313.18];
C = pchip(FZ_C, C_param, abs(FZ));

% Basic Coefficients
kx = (A1 .* (FZ.^2)) + (A2 .* (FZ)) + A3;
mu_x = ((B1 .* (FZ.^2)) + (B2 .* (FZ)) + B3);
mu_y = ((C1 .* (FZ.^3)) + (C2 .* (FZ.^2)) + (C3 .* (FZ)) + C4);

% Normalized Slip Ratio, Slip Angle
s_bar = (kx .* SL) ./ (mu_x .* FZ);

% C is a function of FZ, but it is not an analytical expression
a_bar = (C .* tan(SA)) ./ (mu_y .* FZ);

% Combined Slip Model Parameters
n0 = (C .* mu_x) ./ (kx .* mu_y);
k = sqrt(s_bar.^2 + a_bar.^2);
n = [1 1 1 1];

for i = 1:4
    if abs(k(i)) <= (2*pi)
       n = (0.5 .* (1 + n0)) - (0.5 .* cos(k/2) .* (1 - n0));
    end
end

% Compute R, the bridge between tire slip and tire forces
R = (a .* exp(b .* k)) + (c .* exp(d .* k));

% Find FX & FY, denominator blows up at no slip
FY = [0 0 0 0];

for i = 1:4
   if (abs(SL(i)) == 0.001) && ((abs(SA(i)) == 0.1) || abs(n(i)) < 0.001)
       FY(i) = 0;
   elseif (sqrt(SL(i).^2 + ((n(i).^2) .* (tan(SA(i))).^2))) < 0.001
       FY(i) = 0;
   else
%        FX(i) = (mu_x(i) .* FZ(i) .* R(i) .* SL(i)) ./ (sqrt(SL(i).^2 + ((n(i).^2) .* (tan(SA(i))).^2)));
       FY(i) = (n(i) .* R(i) .* tan(SA(i)) .* mu_y(i) .* FZ(i)) ./ (sqrt(SL(i).^2 + ((n(i).^2) .* (tan(SA(i))).^2)));
   end
end


%% Max Longitudinal Force
% Constant during runtime
R_max = [1 1 1 1] .* (a .* exp(b .* k_limit)) + (c .* exp(d .* k_limit));
n_max = [1 1 1 1];
if abs(k(i)) <= (2*pi)
   n_max = [1 1 1 1] .* (0.5 .* (1 + n0)) - (0.5 .* cos(k_limit/2) .* (1 - n0));
end

s_bar_max = [0 0 0 0];

for i = 1:4
    if k_limit > abs(a_bar(i))
        s_bar_max(i) = sqrt(k_limit^2 - a_bar(i)^2);
    end
end

SL_max = (s_bar_max .* mu_x .* FZ) ./ (kx);

Fx_max = (mu_factor .* mu_x .* FZ .* R_max .* SL_max) ./ (sqrt(SL_max.^2 + ((n_max.^2) .* (tan(SA)).^2)));

%% Compare FY Calculations
% Incomplete, or will not be implemented
FY = FY .* mu_factor;

end

== matlab function Vehicle_Model_Controller_Mar18/Electric Vehicle Model/MATLAB Function ==
  data: steering_angles input; FY input; FwF output size=[2 2]; FX input; FwR output size=[2 2]
function [FwF, FwR] = fcn(steering_angles, FY, FX)
%% Force Transformation, Tire Coordinates to Vehicle Coordinates
FX_FL  = (FX(1) .* cosd(steering_angles)) - (FY(1) .* sind(steering_angles));
FX_FR  = (FX(2) .* cosd(steering_angles)) - (FY(2) .* sind(steering_angles));

FY_FL = (FX(1) .* sind(steering_angles)) + (FY(1) .* cosd(steering_angles));
FY_FR = (FX(2) .* sind(steering_angles)) + (FY(2) .* cosd(steering_angles));


%% Construct Force Matrix
FwF = [[FX_FL; FX_FR] [FY_FL; FY_FR]];
FwR = [FX(3:4) FY(3:4)];
